simulink model "Serial_In_2015"  (R2015a)
settings: Solver=ode45  SolverMode=SingleTasking  StartTime=0.0  StopTime=inf  RelTol=1e-3
libraries: instrumentlib x1
settings Model: SimulationMode=accelerator  CovMetricSettings=dwe  CovHtmlReporting=off  covSaveCumulativeToWorkspaceVar=off  CovSaveSingleToWorkspaceVar=off  CovExternalEMLEnable=on  Creator=LuisFernando  LastModifiedBy=LuisFernando
settings DataIOCC: LimitDataPoints=off  SaveFormat=Dataset
settings OptimizationCC: EfficientMapNaN2IntZero=off
settings DebuggingCC: SFUnexpectedBacktrackingDiag=error  SFNoUnconditionalDefaultTransitionDiag=error
settings HardwareCC: ProdBitPerPointer=64  ProdLargestAtomicFloat=Float  ProdIntDivRoundTo=Zero  ProdEndianess=LittleEndian  ProdHWDeviceType=Specified  TargetBitPerPointer=64  TargetLongLongMode=on  TargetIntDivRoundTo=Zero  TargetEndianess=LittleEndian  TargetWordSize=64  TargetHWDeviceType=MATLAB Host  ProdEqTarget=off
settings ModelReferenceCC: PropagateSignalLabelsOutOfModel=on
settings CodeAppCC: MaxIdLength=128
settings GRTTargetCC: GeneratePreprocessorConditionals=Use local settings  CombineOutputUpdateFcns=off  GRTInterface=on

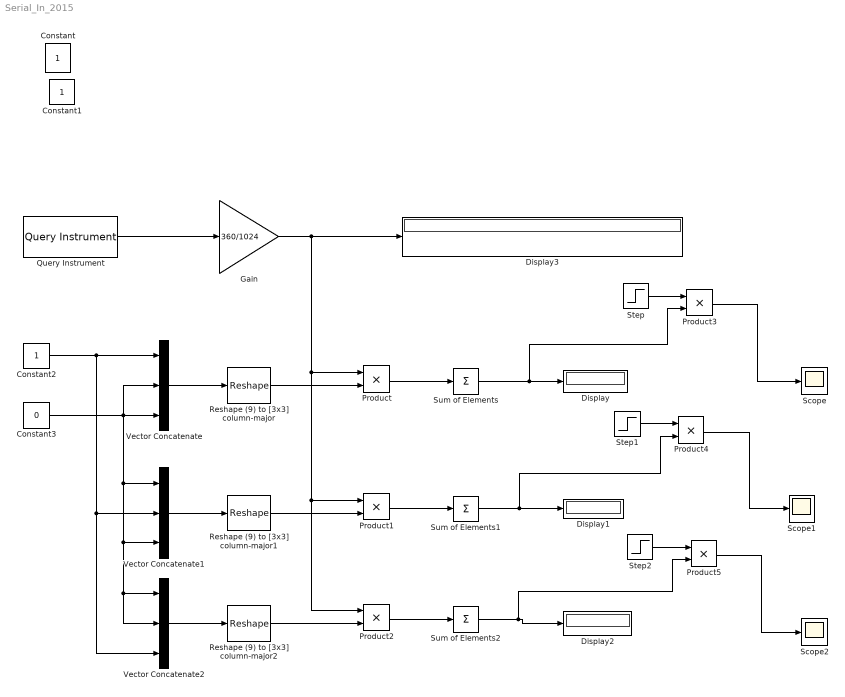
== system Serial_In_2015 ==
  Constant2 : Constant
  Constant3 : Constant  Value=0
  Display{,1..3} (4 alike) : Display
  Gain : Gain  Gain=360/1024
  Product{,1..5} (6 alike) : Product
  Query Instrument : instrumentlib/Query Instrument  sampleTime=100  isWorkspaceObject=off  timeout=1  inputBufferSize=1000  protocol=Serial  serialPort=COM4  baudRate=9600  gpibVendor=Agilent Technologies  boardIndex=0  primaryAddress=1  secondaryAddress=0  visaVendor=Agilent  visaSerialPort=0  chassisIndex=0  logicalAddress=0  tcpRemoteHost='127.0.0.1'  tcpRemotePort=4500  udpRemoteHost='127.0.0.1'  udpRemotePort=9090  visaTCPBoardIndex=0  visaTCPRemoteHost='127.0.0.1'  usbBoardIndex=0  usbManufID=0  usbModelCode=0  usbSerialNumber=0  wsVariableName=puerto  initAction=None  initCommand='DATA:SOURCE CH1'  initFunction=get  queryCommand='1r'  responseFormat=ASCII  asciiFormatting=',%d,%d,%dr'  precision=8-bit integer  byteOrder=Little endian  valuesToRead=1  removeBytes=off  afterOutputAction=Repeat query for new data  enableFrames=on  frameSize=3
  Reshape (9) to [3x3] column-major : Reshape  OutputDimensionality=Column vector (2-D)  OutputDimensions=[1,3]
  Reshape (9) to [3x3] column-major1 : Reshape  OutputDimensionality=Column vector (2-D)  OutputDimensions=[1,3]
  Reshape (9) to [3x3] column-major2 : Reshape  OutputDimensionality=Column vector (2-D)  OutputDimensions=[1,3]
  Scope : Scope
      settings: TimeRange=auto  LimitDataPoints=on  MaxDataPoints=5000  SaveToWorkspace=off  SaveName=ScopeData  YMin=0  YMax=360  SampleTime=-1
  Scope1 : Scope
      settings: TimeRange=auto  LimitDataPoints=on  MaxDataPoints=5000  SaveToWorkspace=off  YMin=260.35156  YMax=460.35156  SampleTime=-1
  Scope2 : Scope
      settings: TimeRange=auto  LimitDataPoints=on  MaxDataPoints=5000  SaveToWorkspace=off  SaveName=ScopeData2  YMin=260.35156  YMax=460.35156  SampleTime=-1
  Step : Step  Time=0.01  SampleTime=0
  Step1 : Step  Time=0.01  SampleTime=0
  Step2 : Step  Time=0.01  SampleTime=0
  Sum of Elements : Sum  Inputs=+
  Sum of Elements1 : Sum  Inputs=+
  Sum of Elements2 : Sum  Inputs=+
  Vector Concatenate : Concatenate  NumInputs=3
  Vector Concatenate1 : Concatenate  NumInputs=3
  Vector Concatenate2 : Concatenate  NumInputs=3
  Constant : Constant  IOType=siggen  VectorParams1D=off  SampleTime=1
  Constant1 : Constant  IOType=siggen
  wires:
  Vector Concatenate/1 -> Reshape (9) to [3x3] column-major/1
  Constant3/1 -> Vector Concatenate2/1, Vector Concatenate2/2, Vector Concatenate1/3, Vector Concatenate1/1, Vector Concatenate/2, Vector Concatenate/3
  Vector Concatenate1/1 -> Reshape (9) to [3x3] column-major1/1
  Vector Concatenate2/1 -> Reshape (9) to [3x3] column-major2/1
  Constant2/1 -> Vector Concatenate2/3, Vector Concatenate1/2, Vector Concatenate/1
  Query Instrument/1 -> Gain/1
  Reshape (9) to [3x3] column-major/1 -> Product/2
  Reshape (9) to [3x3] column-major2/1 -> Product2/2
  Reshape (9) to [3x3] column-major1/1 -> Product1/2
  Gain/1 -> Product1/1, Product2/1, Product/1, Display3/1
  Product/1 -> Sum of Elements/1
  Product1/1 -> Sum of Elements1/1
  Product2/1 -> Sum of Elements2/1
  Sum of Elements/1 -> Product3/2, Display/1
  Step/1 -> Product3/1
  Product3/1 -> Scope/1
  Sum of Elements1/1 -> Product4/2, Display1/1
  Product4/1 -> Scope1/1
  Step1/1 -> Product4/1
  Sum of Elements2/1 -> Product5/2, Display2/1
  Product5/1 -> Scope2/1
  Step2/1 -> Product5/1
